simulink model "main_model"  (R2022a)
settings: Solver=VariableStepAuto  StartTime=0.0  StopTime=10.0  RelTol=1e-3
libraries: visionsources x2
settings Model: Creator=DASARI SUDHEERA  LastModifiedBy=DASARI SUDHEERA

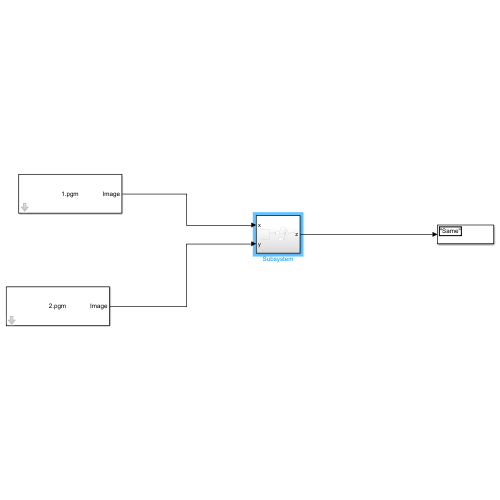
[thumbnail: Simulink's stored preview of the top-level diagram]
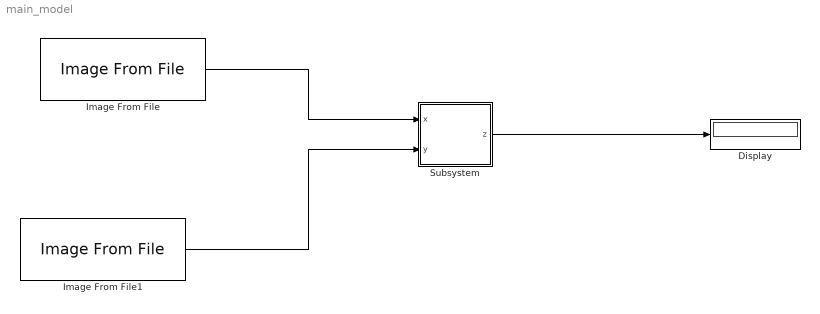
== system main_model ==
  Display : Display
  Image From File : visionsources/Image From File  Tag=vipblks_nd  FileName=D:\Dataset\s1\1.pgm  Ts=inf  imagePorts=One multidimensional signal  OutPortLabels=R|G|B  ImageDataType=Inherit from input image  sdImageDataType=uint(8)  Signed=on  WordLength=16  FractionLengthMode=User-defined  FractionLength=15
  Image From File1 : visionsources/Image From File  Tag=vipblks_nd  FileName=D:\Dataset\s1\2.pgm  Ts=inf  imagePorts=One multidimensional signal  OutPortLabels=R|G|B  ImageDataType=Inherit from input image  sdImageDataType=uint(8)  Signed=on  WordLength=16  FractionLengthMode=User-defined  FractionLength=15
  Subsystem : Subsystem
  wires:
  Image From File/1 -> Subsystem/1(x)
  Image From File1/1 -> Subsystem/2(y)
  Subsystem/1(z) -> Display/1

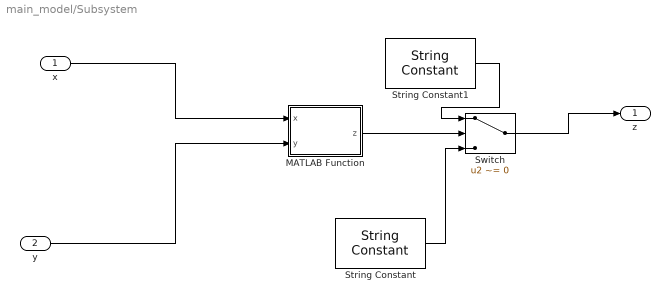
== system main_model/Subsystem ==
  x : Inport
  y : Inport  Port=2
  MATLAB Function : MATLAB Function  TreatAsAtomicUnit=on
  String Constant : StringConstant  String="\"Same\""
  String Constant1 : StringConstant  String="\"Different\""
  Switch : Switch  Criteria=u2 ~= 0  SaturateOnIntegerOverflow=off  InputSameDT=off
  z : Outport
  wires:
  x/1 -> MATLAB Function/1(x)
  y/1 -> MATLAB Function/2(y)
  MATLAB Function/1(z) -> Switch/2
  String Constant/1 -> Switch/3
  String Constant1/1 -> Switch/1
  Switch/1 -> z/1

== matlab function main_model/Subsystem/MATLAB Function ==
  data: x input; z output; y input
function z = fcn(x,y)
g=size(x);
y=imresize(y,[g(1),g(2)]);
figure;
if(x==y)
    z=1;
else
    z=0;
end
